simulink model "Observador"  (R2023b)
settings: Solver=VariableStepAuto  StartTime=0.0  StopTime=10.0  RelTol=1e-3
values from neighbouring files (symbols this model uses):
  A = sym(zeros(7,7))    [Analisis_Contr_Obs.m]    (also in Gs_simbolica.m; Modelo_SS.m = zeros(7,7))
  Bc = sym(zeros(7,1))    [Analisis_Contr_Obs.m]    (also in Modelo_SS.m = zeros(7,1))
  C_s = [0 1 0 0 0 0 0]    [Modelo_SS.m]
undefined symbols (not defined in the file or in its folder): L, L_i
settings Model: Creator=rodri  LastModifiedBy=rodri

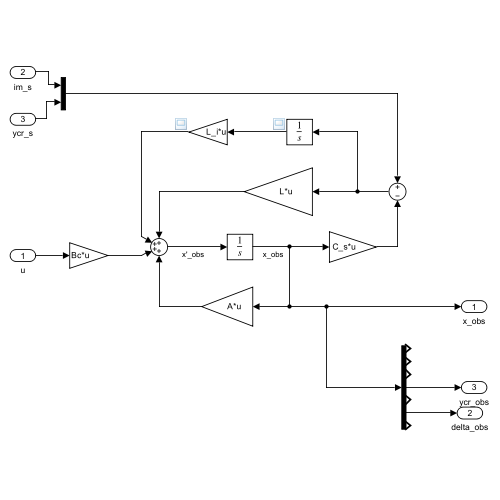
[thumbnail: Simulink's stored preview of the top-level diagram]
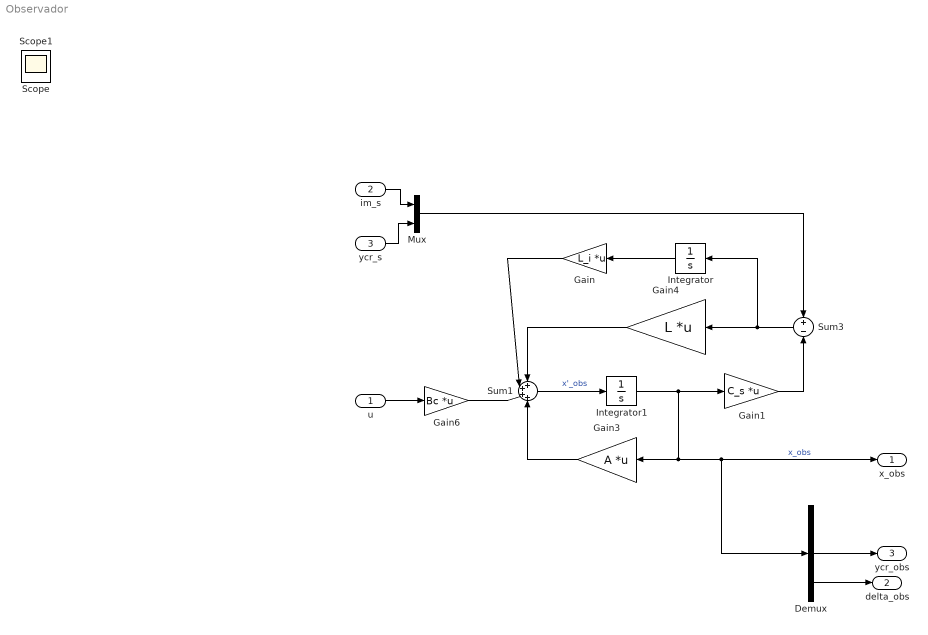
== system Observador ==
  u : Inport
  im_s : Inport  Port=2
  ycr_s : Inport  Port=3
  Demux : Demux  Outputs=7
  Gain : Gain  Gain=L_i  Multiplication=Matrix(K*u)
  Gain1 : Gain  Gain=C_s  Multiplication=Matrix(K*u)
  Gain3 : Gain  Gain=A  Multiplication=Matrix(K*u)
  Gain4 : Gain  Gain=L  Multiplication=Matrix(K*u)
  Gain6 : Gain  Gain=Bc  Multiplication=Matrix(K*u)
  Integrator : Integrator
  Integrator1 : Integrator
  Mux : Mux  Inputs=2
  Sum1 : Sum  Inputs=++++
  Sum3 : Sum  Inputs=+|-
  x_obs : Outport  VectorParamsAs1DForOutWhenUnconnected=off
  delta_obs : Outport  Port=2  VectorParamsAs1DForOutWhenUnconnected=off
  ycr_obs : Outport  Port=3  VectorParamsAs1DForOutWhenUnconnected=off
  Scope : Scope
  Scope1 : Scope
  wires:
  Sum1/1 -> Integrator1/1  "x'_obs"
  Gain1/1 -> Sum3/2
  Integrator1/1 -> Demux/1, x_obs/1, Gain3/1, Gain1/1  "x_obs"
  Sum3/1 -> Integrator/1, Gain4/1
  u/1 -> Gain6/1
  Gain4/1 -> Sum1/1
  Gain3/1 -> Sum1/4
  im_s/1 -> Mux/1
  ycr_s/1 -> Mux/2
  Mux/1 -> Sum3/1
  Demux/6 -> delta_obs/1
  Demux/4 -> ycr_obs/1
  Integrator/1 -> Gain/1
  Gain6/1 -> Sum1/3
  Gain/1 -> Sum1/2
